simulink model "Trabajo3_control_real_estado_Kalman"  (R2024b)
settings: Solver=ode45  StartTime=0.0  StopTime=tmax  MaxStep=0.01  RelTol=1e-3  EnableMultiTasking=on
undefined symbols (not defined in the file): Beta, c, CI, K, Mu, pert, Ts, V, x0, Y0
libraries: simulink x1
settings Model: Creator=CarlosM  LastModifiedBy=Juanj
settings SolverCC: AlgebraicLoopSolver=TrustRegion
settings DataIOCC: SaveFormat=Array  SaveOutput=off  SignalLogging=off  DSMLogging=off  SaveTime=off  ReturnWorkspaceOutputs=off
settings OptimizationCC: ReuseModelBlockBuffer=off  LifeSpan=inf
settings DebuggingCC: UnderspecifiedInitializationDetection=Classic  MergeDetectMultiDrivingBlocksExec=none  SolverPrmCheckMsg=warning  UnconnectedInputMsg=warning  UnconnectedOutputMsg=warning  UnconnectedLineMsg=warning  StateNameClashWarn=warning  SFUnexpectedBacktrackingDiag=warning  SFNoUnconditionalDefaultTransitionDiag=warning  SFExecutionAtInitializationDiag=none  ArithmeticOperatorsInVariantConditions=warning
settings HardwareCC: ProdBitPerPointer=32  ProdBitPerSizeT=32  ProdBitPerPtrDiffT=32  ProdLargestAtomicFloat=None  ProdIntDivRoundTo=Undefined  ProdEndianess=Unspecified  ProdWordSize=32  ProdHWDeviceType=32-bit Generic
settings ModelReferenceCC: EnableRefExpFcnMdlSchedulingChecks=on  PropagateSignalLabelsOutOfModel=off
settings SFSimCC: SimUseLocalCustomCode=off  CustomCodeUndefinedFunction=UseInterfaceOnly
settings RTWCC: RTWUseLocalCustomCode=off  GPUComputeCapability=3.5  DLArmComputeVersion=19.05
settings CodeAppCC: StateflowObjectComments=on
settings GRTTargetCC: TargetLangStandard=C89/C90 (ANSI)
settings ConfigComp: CovMetricSettings=dw  CovSaveCumulativeToWorkspaceVar=on  CovSaveSingleToWorkspaceVar=on  CovExternalEMLEnable=off

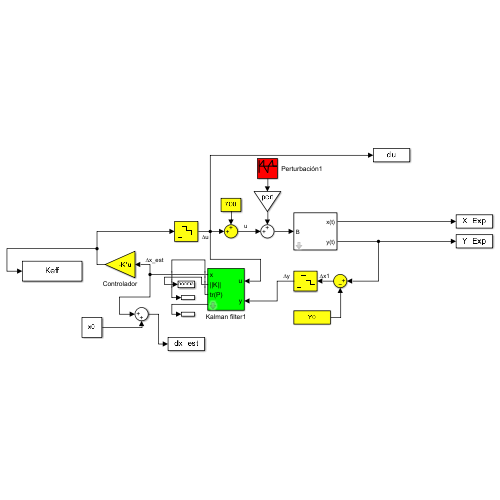
[thumbnail: Simulink's stored preview of the top-level diagram]
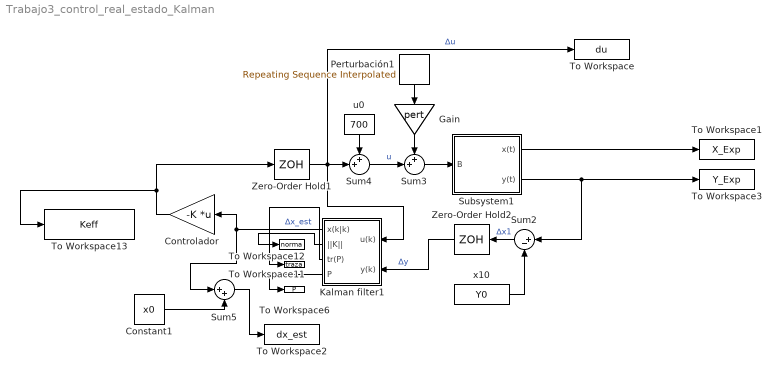
== system Trabajo3_control_real_estado_Kalman ==
  Constant1 : Constant  Value=x0
  Controlador : Gain  Gain=-K  Multiplication=Matrix(K*u)
  Gain : Gain  Gain=pert
  Kalman filter1 : Subsystem  mask(Filtro de Kalman lineal){Sd={Fi, Gamma, C}, xu0=x0, P0QR={P0  Q R}, Ts=Ts}
      mask prompts: Sd "{A,B,C} - Discrete-time system model"; xu0 "x0 - Initial conditions"; P0QR "{P0,Q,R}"; Ts "Ts - Sample time"
      mask init:
      | A = Sd{1}; B = Sd{2}; C = Sd{3};
      | P0 = P0QR{1}; Q = P0QR{2}; R = P0QR{3};
      mask Display:
      | port_label('input', 1, 'u')
      | port_label('input', 2, 'y')
      | port_label('output', 1, 'x')
      | port_label('output', 2, '||K||')
      | port_label('output', 3, 'tr(P)')
  Perturbación1 : simulink/Sources/Repeating Sequence Interpolated  OutValues="[0, 20, 0,  -20, 0, 20, 0, 0]"  TimeValues=[0, 500, 510, 1000, 1010, 1500, 1510, 2000]  LookUpMeth=Interpolation-Use End Values  tsamp=-1  OutMin=[]  OutMax=[]  OutDataTypeStr=double  OutputDataTypeScalingMode=double  OutDataType=fixdt(0,8)  OutScaling=2^-10
  Subsystem1 : Subsystem  mask{Beta=Beta, Mu=Mu, V=V, c=c, X0=CI}
      mask prompts: Beta "Tasa de Transmisión (Beta)"; Mu "Tasa de Muertes (Mu)"; V "Tasa de Recuperación (V)"; c "Contactos Suceptibles-Infectados (c)"; X0 "Suceptibles Iniciales (X0)"
  Sum2 : Sum  Inputs=|+-
  Sum3 : Sum  Inputs=++|
  Sum4 : Sum  Inputs=++|
  Sum5 : Sum  Inputs=|++
  To Workspace : ToWorkspace  VariableName=du  SaveFormat=Structure With Time  SampleTime=Ts
  To Workspace1 : ToWorkspace  VariableName=X_Exp  SaveFormat=Structure With Time  SampleTime=Ts
  To Workspace11 : ToWorkspace  VariableName=traza  SaveFormat=Structure With Time  SampleTime=-1
  To Workspace12 : ToWorkspace  VariableName=norma  SaveFormat=Structure With Time  SampleTime=-1
  To Workspace13 : ToWorkspace  VariableName=Keff  SaveFormat=Timeseries  SampleTime=-1
  To Workspace2 : ToWorkspace  VariableName=dx_est  SaveFormat=Structure With Time  SampleTime=Ts
  To Workspace3 : ToWorkspace  VariableName=Y_Exp  SaveFormat=Structure With Time  SampleTime=Ts
  To Workspace6 : ToWorkspace  VariableName=P  SaveFormat=Structure With Time  SampleTime=-1
  Zero-Order Hold1 : ZeroOrderHold  SampleTime=Ts
  Zero-Order Hold2 : ZeroOrderHold  SampleTime=Ts
  u0 : Constant  Value=700
  x10 : Constant  Value=Y0
  wires:
  Controlador/1 -> To Workspace13/1, Zero-Order Hold1/1
  Kalman filter1/1(x(k|k)) -> Controlador/1, Sum5/1  "∆x_est"
  Sum2/1 -> Zero-Order Hold2/1  "∆x1"
  Gain/1 -> Sum3/1
  Perturbación1/1 -> Gain/1
  Sum4/1 -> Sum3/2  "u"
  Subsystem1/1(x(t)) -> To Workspace1/1
  Subsystem1/2(y(t)) -> To Workspace3/1, Sum2/1
  Sum3/1 -> Subsystem1/1(B)
  u0/1 -> Sum4/1
  Zero-Order Hold2/1 -> Kalman filter1/2(y(k))  "∆y"
  x10/1 -> Sum2/2
  Zero-Order Hold1/1 -> Kalman filter1/1(u(k)), To Workspace/1, Sum4/2  "∆u"
  Sum5/1 -> To Workspace2/1
  Constant1/1 -> Sum5/2
  Kalman filter1/4(P) -> To Workspace6/1
  Kalman filter1/3(tr(P)) -> To Workspace11/1
  Kalman filter1/2(||K||) -> To Workspace12/1

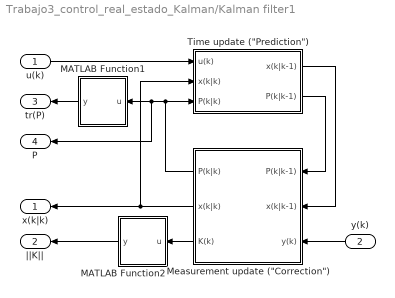
== system Trabajo3_control_real_estado_Kalman/Kalman filter1 ==
  u(k) : Inport
  y(k) : Inport  Port=2
  MATLAB Function1 : MATLAB Function  TreatAsAtomicUnit=on
  MATLAB Function2 : MATLAB Function  TreatAsAtomicUnit=on
  "Measurement update (\"Correction\")" : Subsystem
  "Time update (\"Prediction\")" : Subsystem
  x(k|k) : Outport
  ||K|| : Outport  Port=2
  tr(P) : Outport  Port=3
  P : Outport  Port=4
  wires:
  MATLAB Function1/1(y) -> tr(P)/1
  MATLAB Function2/1(y) -> ||K||/1
  "Measurement update (\"Correction\")"/3(K(k)) -> MATLAB Function2/1(u)
  u(k)/1 -> "Time update (\"Prediction\")"/1(u(k))
  y(k)/1 -> "Measurement update (\"Correction\")"/3(y(k))
  "Time update (\"Prediction\")"/2(P(k|k-1)) -> "Measurement update (\"Correction\")"/1(P(k|k-1))
  "Time update (\"Prediction\")"/1(x(k|k-1)) -> "Measurement update (\"Correction\")"/2(x(k|k-1))
  "Measurement update (\"Correction\")"/2(x(k|k)) -> "Time update (\"Prediction\")"/2(x(k|k)), x(k|k)/1
  "Measurement update (\"Correction\")"/1(P(k|k)) -> "Time update (\"Prediction\")"/3(P(k|k)), P/1, MATLAB Function1/1(u)

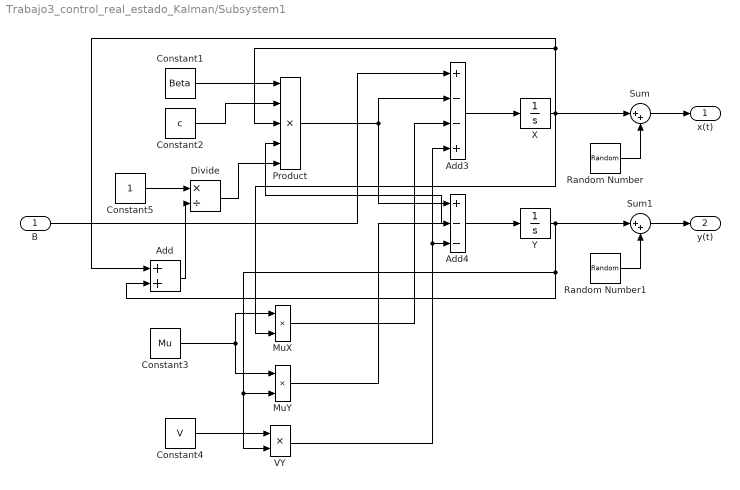
== system Trabajo3_control_real_estado_Kalman/Subsystem1 ==
  B : Inport
  Add : Sum
  Add3 : Sum  Inputs=+--+
  Add4 : Sum  Inputs=+--
  Constant1 : Constant  Value=Beta
  Constant2 : Constant  Value=c
  Constant3 : Constant  Value=Mu
  Constant4 : Constant  Value=V
  Constant5 : Constant
  Divide : Product  Inputs=*/
  MuX : Product
  MuY : Product
  Product : Product  Inputs=5
  Random Number : RandomNumber  Variance=64  SampleTime=Ts
  Random Number1 : RandomNumber  Variance=640  SampleTime=Ts
  Sum : Sum  Inputs=|++
  Sum1 : Sum  Inputs=|++
  VY : Product
  X : Integrator  InitialCondition=X0(1)  LimitOutput=on  LowerSaturationLimit=0
  Y : Integrator  InitialCondition=X0(2)  LimitOutput=on  LowerSaturationLimit=0
  x(t) : Outport
  y(t) : Outport  Port=2
  wires:
  X/1 -> Sum/1, Add/1, Product/3, MuX/2
  MuY/1 -> Add4/2
  Divide/1 -> Product/5
  Y/1 -> Sum1/1, Add/2, MuY/2, VY/2, Product/4
  Constant1/1 -> Product/1
  MuX/1 -> Add3/3
  Constant4/1 -> VY/1
  Add3/1 -> X/1
  Product/1 -> Add4/1, Add3/2
  Constant3/1 -> MuX/1, MuY/1
  B/1 -> Add3/1
  Add4/1 -> Y/1
  Constant2/1 -> Product/2
  Constant5/1 -> Divide/1
  VY/1 -> Add4/3, Add3/4
  Add/1 -> Divide/2
  Random Number/1 -> Sum/2
  Sum/1 -> x(t)/1
  Random Number1/1 -> Sum1/2
  Sum1/1 -> y(t)/1

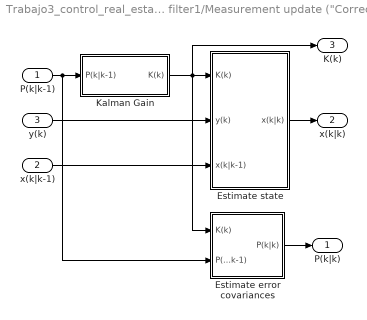
== system Trabajo3_control_real_estado_Kalman/Kalman filter1/Measurement update ("Correction") ==
  P(k|k-1) : Inport
  x(k|k-1) : Inport  Port=2
  y(k) : Inport  Port=3
  Estimate error covariances : Subsystem
  Estimate state : Subsystem
  Kalman Gain : Subsystem
  P(k|k) : Outport
  x(k|k) : Outport  Port=2
  K(k) : Outport  Port=3
  wires:
  P(k|k-1)/1 -> Kalman Gain/1(P(k|k-1)), Estimate error covariances/2(P(k|k-1))
  Kalman Gain/1(K(k)) -> Estimate state/1(K(k)), Estimate error covariances/1(K(k)), K(k)/1
  y(k)/1 -> Estimate state/2(y(k))
  Estimate state/1(x(k|k)) -> x(k|k)/1
  Estimate error covariances/1(P(k|k)) -> P(k|k)/1
  x(k|k-1)/1 -> Estimate state/3(x(k|k-1))

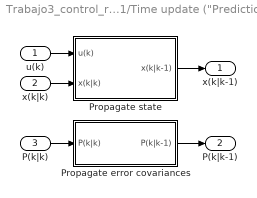
== system Trabajo3_control_real_estado_Kalman/Kalman filter1/Time update ("Prediction") ==
  u(k) : Inport
  x(k|k) : Inport  Port=2
  P(k|k) : Inport  Port=3
  Propagate error covariances : Subsystem
  Propagate state : Subsystem
  x(k|k-1) : Outport
  P(k|k-1) : Outport  Port=2
  wires:
  u(k)/1 -> Propagate state/1(u(k))
  Propagate state/1(x(k|k-1)) -> x(k|k-1)/1
  x(k|k)/1 -> Propagate state/2(x(k|k))
  P(k|k)/1 -> Propagate error covariances/1(P(k|k))
  Propagate error covariances/1(P(k|k-1)) -> P(k|k-1)/1

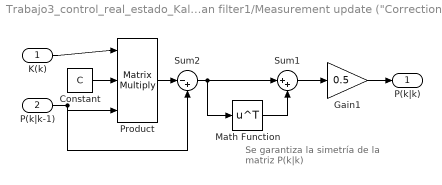
== system Trabajo3_control_real_estado_Kalman/Kalman filter1/Measurement update ("Correction")/Estimate error covariances ==
  note: Se garantiza la simetría
      | de la matriz P(k|k)
  K(k) : Inport
  P(k|k-1) : Inport  Port=2
  Constant : Constant  Value=C  VectorParams1D=off  SampleTime=Ts
  Gain1 : Gain  Gain=0.5
  Math Function : Math  Operator=transpose  SignedPower=on
  Product : Product  Inputs=3  Multiplication=Matrix(*)
  Sum1 : Sum  Inputs=|++
  Sum2 : Sum  Inputs=|-+
  P(k|k) : Outport
  wires:
  Constant/1 -> Product/2
  Product/1 -> Sum2/1
  K(k)/1 -> Product/1
  P(k|k-1)/1 -> Sum2/2, Product/3
  Gain1/1 -> P(k|k)/1
  Sum2/1 -> Math Function/1, Sum1/1
  Math Function/1 -> Sum1/2
  Sum1/1 -> Gain1/1

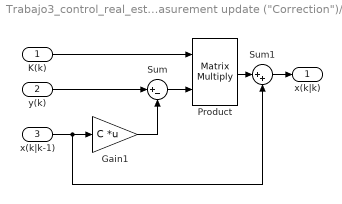
== system Trabajo3_control_real_estado_Kalman/Kalman filter1/Measurement update ("Correction")/Estimate state ==
  K(k) : Inport
  y(k) : Inport  Port=2
  x(k|k-1) : Inport  Port=3
  Gain1 : Gain  Gain=C  Multiplication=Matrix(K*u)
  Product : Product  Multiplication=Matrix(*)
  Sum : Sum  Inputs=|+-
  Sum1 : Sum  Inputs=|++
  x(k|k) : Outport
  wires:
  x(k|k-1)/1 -> Sum1/2, Gain1/1
  Gain1/1 -> Sum/2
  Sum/1 -> Product/2
  Product/1 -> Sum1/1
  K(k)/1 -> Product/1
  Sum1/1 -> x(k|k)/1
  y(k)/1 -> Sum/1

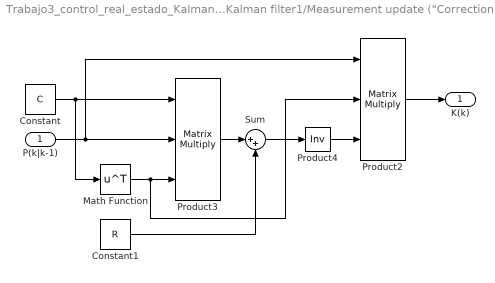
== system Trabajo3_control_real_estado_Kalman/Kalman filter1/Measurement update ("Correction")/Kalman Gain ==
  P(k|k-1) : Inport
  Constant : Constant  Value=C  VectorParams1D=off  SampleTime=Ts
  Constant1 : Constant  Value=R  SampleTime=Ts
  Math Function : Math  Operator=transpose  SignedPower=on
  Product2 : Product  Inputs=3  Multiplication=Matrix(*)
  Product3 : Product  Inputs=3  Multiplication=Matrix(*)
  Product4 : Product  Inputs=/  Multiplication=Matrix(*)
  Sum : Sum  Inputs=|++
  K(k) : Outport
  wires:
  Constant/1 -> Math Function/1, Product3/1
  P(k|k-1)/1 -> Product3/2, Product2/1
  Math Function/1 -> Product3/3, Product2/2
  Product3/1 -> Sum/1
  Constant1/1 -> Sum/2
  Sum/1 -> Product4/1
  Product4/1 -> Product2/3
  Product2/1 -> K(k)/1

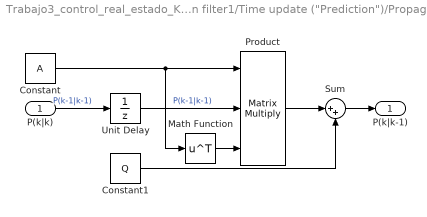
== system Trabajo3_control_real_estado_Kalman/Kalman filter1/Time update ("Prediction")/Propagate error covariances ==
  P(k|k) : Inport
  Constant : Constant  Value=A  SampleTime=Ts
  Constant1 : Constant  Value=Q  SampleTime=Ts
  Math Function : Math  Operator=transpose  SignedPower=on
  Product : Product  Inputs=3  Multiplication=Matrix(*)  RndMeth=Zero  SampleTime=Ts
  Sum : Sum  Inputs=|++
  Unit Delay : UnitDelay  InitialCondition=P0  SampleTime=Ts  HasFrameUpgradeWarning=on
  P(k|k-1) : Outport
  wires:
  P(k|k)/1 -> Unit Delay/1  "P(k-1|k-1)"
  Constant/1 -> Math Function/1, Product/1
  Math Function/1 -> Product/3
  Product/1 -> Sum/1
  Constant1/1 -> Sum/2
  Sum/1 -> P(k|k-1)/1
  Unit Delay/1 -> Product/2  "P(k-1|k-1)"

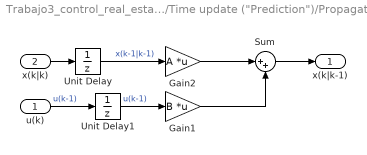
== system Trabajo3_control_real_estado_Kalman/Kalman filter1/Time update ("Prediction")/Propagate state ==
  u(k) : Inport
  x(k|k) : Inport  Port=2
  Gain1 : Gain  Gain=B  Multiplication=Matrix(K*u)
  Gain2 : Gain  Gain=A  Multiplication=Matrix(K*u)
  Sum : Sum  Inputs=|++
  Unit Delay : UnitDelay  InitialCondition=x0  SampleTime=Ts  HasFrameUpgradeWarning=on
  Unit Delay1 : UnitDelay  SampleTime=Ts  HasFrameUpgradeWarning=on
  x(k|k-1) : Outport
  wires:
  Unit Delay/1 -> Gain2/1  "x(k-1|k-1)"
  x(k|k)/1 -> Unit Delay/1
  u(k)/1 -> Unit Delay1/1  "u(k-1)"
  Gain2/1 -> Sum/1
  Gain1/1 -> Sum/2
  Sum/1 -> x(k|k-1)/1
  Unit Delay1/1 -> Gain1/1  "u(k-1)"

== matlab function Trabajo3_control_real_estado_Kalman/Kalman filter1/MATLAB Function2 ==
  data: u input; y output
function y = fcn(u)
y = norm(u);

== matlab function Trabajo3_control_real_estado_Kalman/Kalman filter1/MATLAB Function1 ==
  data: u input; y output
function y = fcn(u)
y = trace(u);
